simulink model "quadPD"  (R2012b)
settings: Solver=ode45  StartTime=0.0  StopTime=Inf  RelTol=1e-3
undefined symbols (not defined in the file or in its folder): sigbuilder_block
libraries: simulink x4, vrlib x1
settings Model: Creator=Estel  LastModifiedBy=Estel

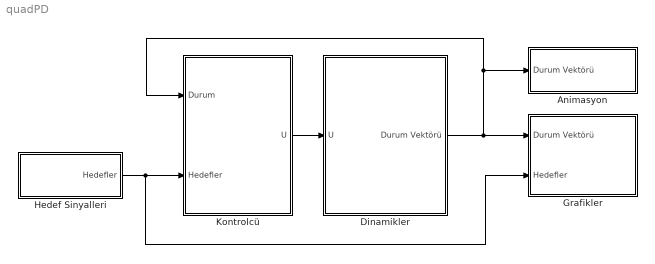
== system quadPD ==
  Animasyon : Subsystem
  Dinamikler : Subsystem
  Grafikler : Subsystem
  Hedef Sinyalleri : Subsystem
  Kontrolcü : Subsystem
  wires:
  Dinamikler/1(Durum Vektörü) -> Animasyon/1(Durum Vektörü), Kontrolcü/1(Durum), Grafikler/1(Durum Vektörü)
  Hedef Sinyalleri/1(Hedefler) -> Grafikler/2(Hedefler), Kontrolcü/2(Hedefler)
  Kontrolcü/1(U) -> Dinamikler/1(U)

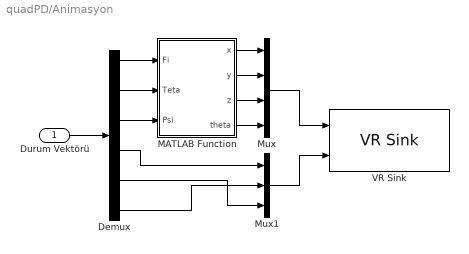
== system quadPD/Animasyon ==
  Durum Vektörü : Inport
  Demux : Demux  Outputs=6
  MATLAB Function : MATLAB Function  TreatAsAtomicUnit=on
  Mux : Mux
  Mux1 : Mux  Inputs=3
  VR Sink : vrlib/VR Sink  InstantiateOnLoad=on  SampleTime=0.1  ViewEnable=on  RemoteChange=off  RemoteView=off  FieldsWritten=Quadro.rotation.4.1.1.double#Quadro.translation.3.1.1.double  WorldFileName=quad.wrl  AutoView=off  VideoDimensions=[]  AllowVariableSize=off
  wires:
  MATLAB Function/2(y) -> Mux/2
  MATLAB Function/4(theta) -> Mux/4
  MATLAB Function/1(x) -> Mux/1
  MATLAB Function/3(z) -> Mux/3
  Mux/1 -> VR Sink/1
  Durum Vektörü/1 -> Demux/1
  Demux/1 -> MATLAB Function/1(Fi)
  Demux/2 -> MATLAB Function/2(Teta)
  Demux/3 -> MATLAB Function/3(Psi)
  Demux/6 -> Mux1/2
  Demux/5 -> Mux1/3
  Demux/4 -> Mux1/1
  Mux1/1 -> VR Sink/2

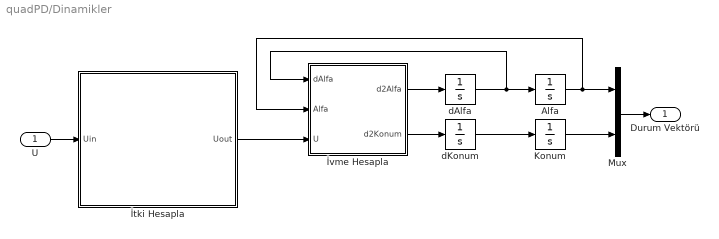
== system quadPD/Dinamikler ==
  U : Inport
  Alfa : Integrator
  Konum : Integrator
  Mux : Mux  Inputs=2
  dAlfa : Integrator
  dKonum : Integrator
  İtki Hesapla : MATLAB Function  TreatAsAtomicUnit=on
  İvme Hesapla : MATLAB Function  TreatAsAtomicUnit=on
  Durum Vektörü : Outport
  wires:
  U/1 -> İtki Hesapla/1(Uin)
  Mux/1 -> Durum Vektörü/1
  İtki Hesapla/1(Uout) -> İvme Hesapla/3(U)
  İvme Hesapla/1(d2Alfa) -> dAlfa/1
  dAlfa/1 -> Alfa/1, İvme Hesapla/1(dAlfa)
  Alfa/1 -> Mux/1, İvme Hesapla/2(Alfa)
  İvme Hesapla/2(d2Konum) -> dKonum/1
  dKonum/1 -> Konum/1
  Konum/1 -> Mux/2

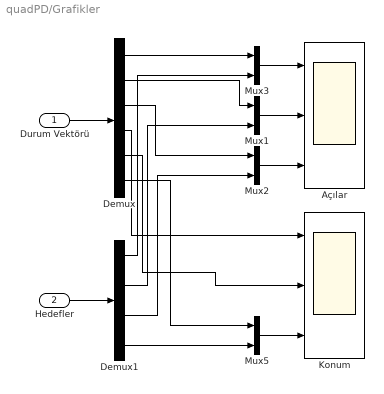
== system quadPD/Grafikler ==
  Durum Vektörü : Inport
  Hedefler : Inport  Port=2
  Açılar : Scope  NumInputPorts=3
      settings: YMin=-25~-5~-5  YMax=550~5~5
  Demux : Demux  Outputs=6
  Demux1 : Demux
  Konum : Scope  NumInputPorts=3
      settings: YMin=-25~-5~-5  YMax=550~5~5  SaveName=ScopeData2
  Mux{1..3,5} (4 alike) : Mux  Inputs=2
  wires:
  Mux2/1 -> Açılar/3
  Mux1/1 -> Açılar/2
  Mux3/1 -> Açılar/1
  Mux5/1 -> Konum/3
  Demux/1 -> Mux3/1
  Demux/2 -> Mux1/1
  Demux/3 -> Mux2/1
  Demux/6 -> Mux5/1
  Demux/4 -> Konum/1
  Demux/5 -> Konum/2
  Demux1/1 -> Mux3/2
  Demux1/2 -> Mux1/2
  Demux1/3 -> Mux2/2
  Demux1/4 -> Mux5/2
  Durum Vektörü/1 -> Demux/1
  Hedefler/1 -> Demux1/1

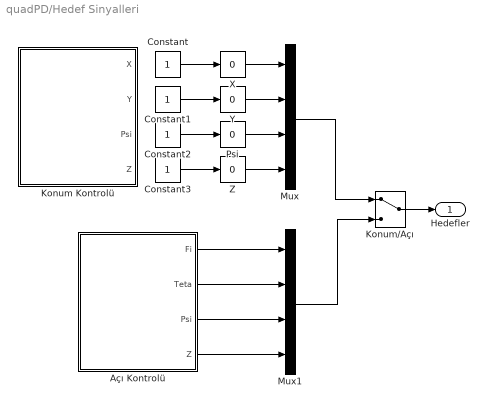
== system quadPD/Hedef Sinyalleri ==
  Açı Kontrolü : Subsystem  Tag=STV Subsys  LoadFcn=sigbuilder_block('load');  StartFcn=sigbuilder_block('start');  StopFcn=sigbuilder_block('stop');  ClipboardFcn=sigbuilder_block('clipboard');  mask(Sigbuilder block){}
      mask help: Simulink:masks:SigbuilderBlock_MD
      mask init:
      | if ~strcmp(get_param(bdroot(gcbh),'SimulationStatus'),'stopped') tuvar = sigbuilder_block('maskInit'); end
      settings: CopyFcn=sigbuilder_block('copy');  DeleteFcn=sigbuilder_block('delete');  ModelCloseFcn=sigbuilder_block('modelClose');  PreSaveFcn=sigbuilder_block('preSave');  PauseFcn=sigbuilder_block('pause');  ContinueFcn=sigbuilder_block('continue');  NameChangeFcn=sigbuilder_block('namechange');  OpenFcn=sigbuilder_block('open',[6 28.5 1012.5 484.5 ]);  CloseFcn=sigbuilder_block('close');
      mask Display: plot(0, 0, 100, 100,[2, 2, 32, 32, 2], [68, 8, 8, 68, 68],[32, 2], [38, 38], [32, 19, 2],[53, 60, 44], [32, 17, 17, 2],[16, 16, 31, 31]);txt = getActiveGroup(gcbh);text(2, 100, txt,'verticalAlignment', 'top');
  Constant{,1..3} (4 alike) : Constant
  Konum Kontrolü : Subsystem  Tag=STV Subsys  LoadFcn=sigbuilder_block('load');  StartFcn=sigbuilder_block('start');  StopFcn=sigbuilder_block('stop');  ClipboardFcn=sigbuilder_block('clipboard');  mask(Sigbuilder block){}
      mask help: Simulink:masks:SigbuilderBlock_MD
      mask init:
      | if ~strcmp(get_param(bdroot(gcbh),'SimulationStatus'),'stopped') tuvar = sigbuilder_block('maskInit'); end
      settings: CopyFcn=sigbuilder_block('copy');  DeleteFcn=sigbuilder_block('delete');  ModelCloseFcn=sigbuilder_block('modelClose');  PreSaveFcn=sigbuilder_block('preSave');  PauseFcn=sigbuilder_block('pause');  ContinueFcn=sigbuilder_block('continue');  NameChangeFcn=sigbuilder_block('namechange');  OpenFcn=sigbuilder_block('open',[6 28.5 1012.5 484.5 ]);  CloseFcn=sigbuilder_block('close');
      mask Display: plot(0, 0, 100, 100,[2, 2, 32, 32, 2], [68, 8, 8, 68, 68],[32, 2], [38, 38], [32, 19, 2],[53, 60, 44], [32, 17, 17, 2],[16, 16, 31, 31]);txt = getActiveGroup(gcbh);text(2, 100, txt,'verticalAlignment', 'top');
  Konum/Açı : ManualSwitch
  Mux : Mux
  Mux1 : Mux
  Psi : simulink/Math Operations/Slider Gain  low=0  gain=0  high=2
  X : simulink/Math Operations/Slider Gain  low=-5  gain=0  high=5
  Y : simulink/Math Operations/Slider Gain  low=-5  gain=0  high=5
  Z : simulink/Math Operations/Slider Gain  low=0  gain=0  high=10
  Hedefler : Outport
  wires:
  Açı Kontrolü/1(Fi) -> Mux1/1
  Açı Kontrolü/2(Teta) -> Mux1/2
  Açı Kontrolü/3(Psi) -> Mux1/3
  Açı Kontrolü/4(Z) -> Mux1/4
  Mux/1 -> Konum/Açı/1
  Mux1/1 -> Konum/Açı/2
  Konum/Açı/1 -> Hedefler/1
  Constant3/1 -> Z/1
  Constant2/1 -> Psi/1
  Constant1/1 -> Y/1
  Constant/1 -> X/1
  Z/1 -> Mux/4
  Psi/1 -> Mux/3
  X/1 -> Mux/1
  Y/1 -> Mux/2

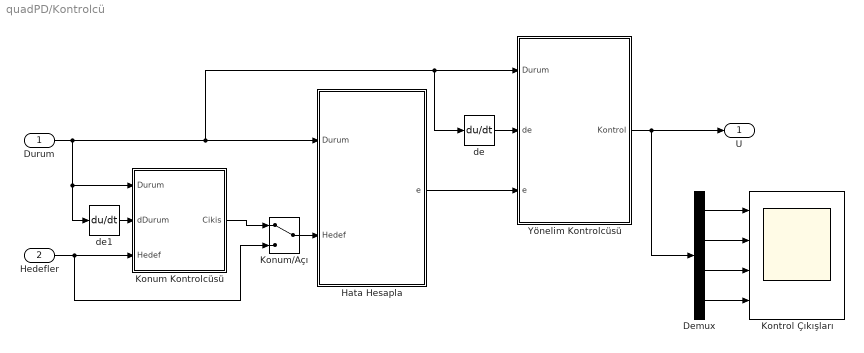
== system quadPD/Kontrolcü ==
  Durum : Inport
  Hedefler : Inport  Port=2
  Demux : Demux
  Hata Hesapla : MATLAB Function  TreatAsAtomicUnit=on
  Kontrol Çıkışları : Scope  NumInputPorts=4
      settings: TimeRange=0.1500000000000004  YMin=-5000000~-160~-195000~1390  YMax=10000000~-154~-180000~1440
  Konum Kontrolcüsü : MATLAB Function  TreatAsAtomicUnit=on
  Konum/Açı : ManualSwitch
  Yönelim Kontrolcüsü : MATLAB Function  TreatAsAtomicUnit=on
  de : Derivative
  de1 : Derivative
  U : Outport
  wires:
  Hedefler/1 -> Konum Kontrolcüsü/3(Hedef), Konum/Açı/2
  Demux/4 -> Kontrol Çıkışları/4
  Demux/3 -> Kontrol Çıkışları/3
  Demux/2 -> Kontrol Çıkışları/2
  Demux/1 -> Kontrol Çıkışları/1
  de/1 -> Yönelim Kontrolcüsü/2(de)
  Hata Hesapla/1(e) -> Yönelim Kontrolcüsü/3(e)
  Yönelim Kontrolcüsü/1(Kontrol) -> U/1, Demux/1
  Durum/1 -> de/1, Yönelim Kontrolcüsü/1(Durum), Hata Hesapla/1(Durum), de1/1, Konum Kontrolcüsü/1(Durum)
  de1/1 -> Konum Kontrolcüsü/2(dDurum)
  Konum/Açı/1 -> Hata Hesapla/2(Hedef)
  Konum Kontrolcüsü/1(Cikis) -> Konum/Açı/1

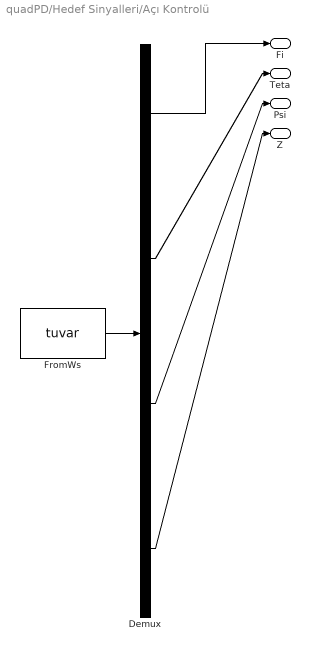
== system quadPD/Hedef Sinyalleri/Açı Kontrolü ==
  Demux : Demux  Tag=STV Demux
  FromWs : FromWorkspace  Tag=STV FromWs  VariableName=tuvar  SampleTime=0
      SigBuilderData=|
      | common.afterFinalStr = 'Extrapolate'
      | common.sampleTime = 0
      | dataSet.timeRange = [0 30]
      | dataSet.name = 'Group 1'
      | sbobj.Groups.Name = 'Group 1'
      | sbobj.Groups.Signals(1).Name = 'Fi'
      | sbobj.Groups.Signals(1).XData = [0 1 1 30]
      | sbobj.Groups.Signals(1).YData = [0 0 1 1]
      | sbobj.Groups.Signals(2).Name = 'Teta'
      | sbobj.Groups.Signals(2).XData = [0 4 4 30]
      | sbobj.Groups.Signals(2).YData = [0 0 1 1]
      | sbobj.Groups.Signals(3).Name = 'Psi'
      | sbobj.Groups.Signals(3).XData = [0 4 6 30]
      | sbobj.Groups.Signals(3).YData = [0 0 0 0]
      | sbobj.Groups.Signals(4).Name = 'Z'
      | sbobj.Groups.Signals(4).XData = [0 4 6 30]
      | sbobj.Groups.Signals(4).YData = [0 0 0 0]
      | sbobj.Groups.TimeRange = [0 30]
  Fi : Outport  Tag=STV Outport
  Teta : Outport  Tag=STV Outport  Port=2
  Psi : Outport  Tag=STV Outport  Port=3
  Z : Outport  Tag=STV Outport  Port=4
  wires:
  Demux/1 -> Fi/1
  FromWs/1 -> Demux/1
  Demux/2 -> Teta/1
  Demux/3 -> Psi/1
  Demux/4 -> Z/1

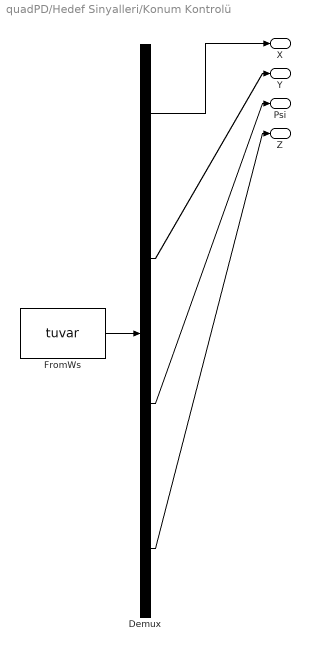
== system quadPD/Hedef Sinyalleri/Konum Kontrolü ==
  Demux : Demux  Tag=STV Demux
  FromWs : FromWorkspace  Tag=STV FromWs  VariableName=tuvar  SampleTime=0
      SigBuilderData=|
      | common.afterFinalStr = 'Extrapolate'
      | common.sampleTime = 0
      | dataSet.timeRange = [0 30]
      | dataSet.name = 'Group 1'
      | sbobj.Groups.Name = 'Group 1'
      | sbobj.Groups.Signals(1).Name = 'X'
      | sbobj.Groups.Signals(1).XData = [0 30]
      | sbobj.Groups.Signals(1).YData = [1 1]
      | sbobj.Groups.Signals(2).Name = 'Y'
      | sbobj.Groups.Signals(2).XData = [0 30]
      | sbobj.Groups.Signals(2).YData = [1 1]
      | sbobj.Groups.Signals(3).Name = 'Psi'
      | sbobj.Groups.Signals(3).XData = [0 4 6 30]
      | sbobj.Groups.Signals(3).YData = [0 0 0 0]
      | sbobj.Groups.Signals(4).Name = 'Z'
      | sbobj.Groups.Signals(4).XData = [0 30]
      | sbobj.Groups.Signals(4).YData = [1 1]
      | sbobj.Groups.TimeRange = [0 30]
  X : Outport  Tag=STV Outport
  Y : Outport  Tag=STV Outport  Port=2
  Psi : Outport  Tag=STV Outport  Port=3
  Z : Outport  Tag=STV Outport  Port=4
  wires:
  Demux/1 -> X/1
  FromWs/1 -> Demux/1
  Demux/2 -> Y/1
  Demux/3 -> Psi/1
  Demux/4 -> Z/1

== matlab function quadPD/Dinamikler/İvme Hesapla ==
  data: dAlfa input; Alfa input; d2Alfa output size=3; U input; d2Konum output size=3
function [d2Alfa, d2Konum]= Ivmeler(dAlfa, Alfa, U)
%#codegen

dFi = dAlfa(1);
dTeta = dAlfa(2);
dPsi = dAlfa(3);
Fi = Alfa(1);
Teta = Alfa(2);
Psi = Alfa(3);
U1 = U(1);
U2 = U(2);
U3 = U(3);
U4 = U(4);
Omega = U(5);

Ixx = 7.5*10^(-3);  % Quadrotor moment of inertia around X axis
Iyy = 7.5*10^(-3);  % Quadrotor moment of inertia around Y axis
Izz = 1.3*10^(-2);  % Quadrotor moment of inertia around Z axis
Jr = 6.5*10^(-5);  % Total rotational moment of inertia around the propeller axis
l = 0.23;  % Distance to the center of the Quadrotor
g = 9.81;   % Gravitational acceleration
m = 0.65;  % Mass of the Quadrotor in Kg

a1 = (Iyy-Izz)/Ixx;
a2 = Jr/Ixx;
a3 = (Izz-Ixx)/Iyy;
a4 = Jr/Iyy;
a5 = (Ixx-Iyy)/Izz;

b1 = l/Ixx;
b2 = l/Iyy;
b3 = l/Izz;

ux = (cos(Fi)*sin(Teta)*cos(Psi)+sin(Fi)*sin(Psi));
uy = (cos(Fi)*sin(Teta)*sin(Psi)-sin(Fi)*cos(Psi));

d2Fi = dTeta*dPsi*a1 + dTeta*a2*Omega + b1*U2;
d2Teta = dFi*dPsi*a3 - dFi*a4*Omega + b2*U3;
d2Psi = dTeta*dFi*a5 + b3*U4;
d2Z = g - (cos(Fi)*cos(Teta))*(1/m)*U1;
d2X = ux*(1/m)*U1;
d2Y = -uy*(1/m)*U1;

d2Alfa = [d2Fi; d2Teta; d2Psi];
d2Konum = [d2X; d2Y; d2Z];

== matlab function quadPD/Dinamikler/İtki Hesapla ==
  data: Uin input size=4; Uout output
function Uout = Itkiler(Uin)
% function [OM_21, OM_22, OM_23, OM_24, OM_2]= fcn(Uin)
%#codegen

U1 = Uin(1);
U2 = Uin(2);
U3 = Uin(3);
U4 = Uin(4);

Ix = 7.5*10^(-3);
Iy = 7.5*10^(-3);
Iz = 1.3*10^(-2);
Jr = 6.5*10^(-5);
b = 3.13*10^(-5);
d = 7.5*10^(-7);
l = 0.23;
m = 0.65;
g = 9.81;

U = [U1 U2 U3 U4];

M = [ 1/(4*b)   0         1/(2*b*l)   -1/(4*d);
      1/(4*b)  -1/(2*b*l)   0          1/(4*d);
      1/(4*b)   0        -1/(2*b*l)   -1/(4*d);
      1/(4*b)   1/(2*b*l)   0          1/(4*d);];
OM_2h = M * U';
OM_2 = OM_2h';

U1_2 = b*(OM_2(1)+OM_2(2)+OM_2(3)+OM_2(4));
U2_2 = b*(-OM_2(2)+OM_2(4));
U3_2 = b*(OM_2(1)-OM_2(3));
U4_2 = d*(-OM_2(1)+OM_2(2)-OM_2(3)+OM_2(4));
Omega = d*(-OM_2(1)+OM_2(2)-OM_2(3)+OM_2(4));

Uout = [U1_2 U2_2 U3_2 U4_2 Omega];

== matlab function quadPD/Kontrolcü/Hata Hesapla ==
  data: Durum input; e output; Hedef input
function e = Hatalar(Durum, Hedef)
%#codegen

FiHedef = Hedef(1);
TetaHedef = Hedef(2);
PsiHedef = Hedef(3);
ZHedef = Hedef(4);
Fi = Durum(1);
Teta = Durum(2);
Psi = Durum(3);
% X = Durum(4);
% Y = Durum(5);
Z = Durum(6);

eFi = FiHedef - Fi;
eTeta = TetaHedef - Teta;
ePsi = PsiHedef - Psi;
eZ = ZHedef - Z;

e = [eZ eFi eTeta ePsi];

== matlab function quadPD/Kontrolcü/Yönelim Kontrolcüsü ==
  data: Durum input; de input; e input; Kontrol output
function Kontrol = YonelimKontrol(Durum, de, e)
%#codegen

eZ = e(1);
eFi = e(2);
eTeta = e(3);
ePsi = e(4);
deFi = de(1);
deTeta = de(2);
dePsi = de(3);
deZ = de(6);
Fi = Durum(1);
Teta = Durum(2);

kpp = 0.8;
kdp = 0.4;
kpt = 1.2;
kdt = 0.4;
kpps = 1;
kdps = 0.4;
kpz = 100;
kdz = 20;
m = 0.65;

Z_kont = 1 - (((eZ*kpz - deZ*kdz)*m)/(cos(Fi)*cos(Teta)));
Fi_kont = (kpp*eFi - kdp*deFi);
Teta_kont = (kpt*eTeta - kdt*deTeta);
Psi_kont = (kpps*ePsi - kdps*dePsi);

Kontrol = [Z_kont Fi_kont Teta_kont Psi_kont];

== matlab function quadPD/Kontrolcü/Konum Kontrolcüsü ==
  data: Durum input; dDurum input; Cikis output; Hedef input
function Cikis = KonumKontrol(Durum, dDurum, Hedef)
%#codegen

Fi = Durum(1);
Teta = Durum(2);
Psi = Durum(3);
X = Durum(4);
Y = Durum(5);
Z = Durum(6);
dX = dDurum(4);
dY = dDurum(5);
XHedef = Hedef(1);
YHedef = Hedef(2);
PsiHedef = Hedef(3);
ZHedef = Hedef(4);

kpx = 0.1;
kdx = 0.15;
kpy = 0.1;
kdy = 0.17;

eX = XHedef - X;
eY = YHedef - Y;

X_kont = (kpx*eX - kdx*dX);
Y_kont = (kpy*eY - kdy*dY);

Cikis = [Y_kont X_kont PsiHedef ZHedef];

== matlab function quadPD/Animasyon/MATLAB Function ==
  data: Fi input; Teta input; x output; Psi input; y output; z output; theta output
function [x, y, z, theta]= euler2axis(Fi, Teta, Psi)
%#codegen

Teta = -Teta;
theta = 2*acos(cos(Psi/2)*cos(Teta/2)*cos(Fi/2)-sin(Psi/2)*sin(Teta/2)*sin(Fi/2));
x = sin(Psi/2)*sin(Teta/2)*cos(Fi/2)+cos(Psi/2)*cos(Teta/2)*sin(Fi/2);
y = sin(Psi/2)*cos(Teta/2)*cos(Fi/2)+cos(Psi/2)*sin(Teta/2)*sin(Fi/2);
z = cos(Psi/2)*sin(Teta/2)*cos(Fi/2)+sin(Psi/2)*cos(Teta/2)*sin(Fi/2);
